simulink library "lib_wheel"  (Simulink 4.1.1)
undefined symbols (not defined in the file or in its folder): veh_mass, wh_axle_loss_mass, wh_axle_loss_trq, wh_front_active_bool, wh_inertia, wh_max_front_brake_force, wh_max_rear_brake_force, wh_radius, wh_rear_active_bool, wh_slip, wh_slip_force_coeff
libraries: lib_wheel x6
(part 1 of 2)
settings Model: LastModifiedBy=tmarkel
settings Model: ModifiedComment=|
  | mokeefe -- Thu Apr 18 08:40:34 2002 -- Version 1.10
  | saving the model:
  | o "without the model browser open"
  | o with only top-level screen visible
  | o with "fit to view" enabled
  | o with "status bar" off and "toolbar" off
  | o with "prompt to update model history with each save" on
settings Model: ModifiedHistory=|
  | mokeefe -- Thu Apr 18 08:40:34 2002 -- Version 1.10
  | saving the model:
  | o "without the model browser open"
  | o with only top-level screen visible
  | o with "fit to view" enabled
  | o with "status bar" off and "toolbar" off
  | o with "prompt to update model history with each save" on
  | 
  | mokeefe -- Thu Apr 18 08:40:34 2002 -- Version 1.10
  | saving the model:
  | o "without the model browser open"
  | o with only top-level screen visible
  | o with "fit to view" enabled
  | o with "status bar" off and "toolbar" off
  | o with "prompt to update model history with each save" on
  | 
  | ssprik -- Fri Feb 01 16:13:25 2002 -- Version 1.9
  | added wheel goto tag wh_trq_a
  | 
  | mokeefe -- Fri Jun 29 14:51:12 2001 -- Version 1.8
  | 
  | added sub-model component to calculate vehicle weight
  | 
  | mokeefe -- Fri Jun 29 14:49:48 2001 -- Version 1.7
  | 
  | 
  | mokeefe -- Thu Jun 28 14:08:49 2001 -- Version 1.6
  | 
  | replaced all 'veh_mass' references with a veh_mass plus a FROM block (originating from drive cycle) that gives variable cargo mass by time

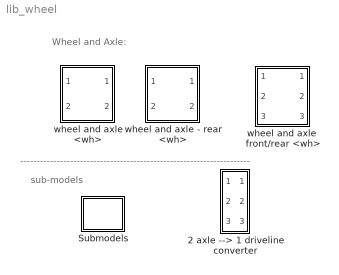
== system lib_wheel ==
  note: Wheel and Axle:
  note: ---------------------------------------------------------------------
  note: sub-models
  2 axle --> 1 driveline converter : Subsystem
      settings: RTWFcnNameOpts=Auto  RTWFileNameOpts=Auto
  Submodels : Subsystem
      settings: RTWFcnNameOpts=Auto  RTWFileNameOpts=Auto
  wheel and axle - rear <wh> : Subsystem
      settings: RTWFcnNameOpts=Auto  RTWFileNameOpts=Auto
      mask Display: image(imread('bdi_wh.jpg'))
  wheel and axle <wh> : Subsystem
      settings: RTWFcnNameOpts=Auto  RTWFileNameOpts=Auto
      mask Display: image(imread('bdi_wh.jpg'))
  wheel and axle  front/rear <wh> : Subsystem
      settings: RTWFcnNameOpts=Auto  RTWFileNameOpts=Auto
      mask Display: image(imread('bdi_wh.jpg'))

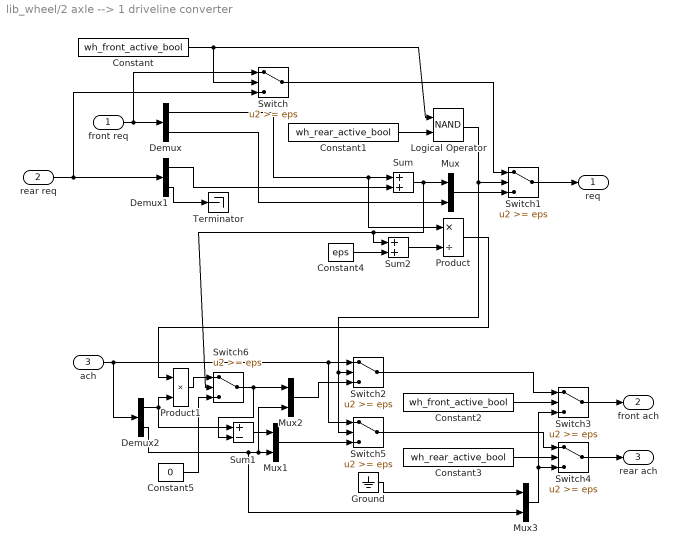
== system lib_wheel/2 axle --> 1 driveline converter ==
  front req : Inport  Port=1  LatchInput=off
  rear req : Inport  Port=2  LatchInput=off
  ach : Inport  Port=3  LatchInput=off
  Constant : Constant  Value=wh_front_active_bool
  Constant1 : Constant  Value=wh_rear_active_bool
  Constant2 : Constant  Value=wh_front_active_bool
  Constant3 : Constant  Value=wh_rear_active_bool
  Constant4 : Constant  Value=eps
  Constant5 : Constant  Value=0
  Demux : Demux  Outputs=2  BusSelectionMode=off
  Demux1 : Demux  Outputs=2  BusSelectionMode=off
  Demux2 : Demux  Outputs=2  BusSelectionMode=off
  Ground : Ground
  Logical Operator : Logic  Operator=NAND  Inputs=2
  Mux{,1..3} (4 alike) : Mux  Inputs=2
  Product : Product  Inputs=*/  Multiplication=Element-wise(.*)  SaturateOnIntegerOverflow=on
  Product1 : Product  Inputs=2  Multiplication=Element-wise(.*)  SaturateOnIntegerOverflow=on
  Sum : Sum  Inputs=++  SaturateOnIntegerOverflow=on
  Sum1 : Sum  Inputs=+-  SaturateOnIntegerOverflow=on
  Sum2 : Sum  Inputs=++  SaturateOnIntegerOverflow=on
  Switch{,1..6} (7 alike) : Switch  Threshold=eps
  Terminator : Terminator
  req : Outport  Port=1
  front ach : Outport  Port=2
  rear ach : Outport  Port=3
  wires:
  rear req/1 -> Demux1/1, Switch/3
  Constant/1 -> Switch/2, Logical Operator/1
  Switch/1 -> Switch1/1
  Logical Operator/1 -> Switch1/2, Switch2/2, Switch5/2
  Switch1/1 -> req/1
  Mux/1 -> Switch1/3
  Demux1/1 -> Sum/2
  Demux/1 -> Sum/1, Product/1
  Sum/1 -> Mux/1, Sum2/1, Switch6/2
  Demux/2 -> Mux/2
  Demux1/2 -> Terminator/1
  front req/1 -> Demux/1, Switch/1
  Constant1/1 -> Logical Operator/2
  ach/1 -> Demux2/1, Switch2/1, Switch5/1
  Switch3/1 -> front ach/1
  Switch4/1 -> rear ach/1
  Demux2/1 -> Product1/2, Sum1/1
  Product/1 -> Product1/1
  Sum1/1 -> Mux1/1
  Constant3/1 -> Switch4/2
  Constant2/1 -> Switch3/2
  Ground/1 -> Mux3/1
  Mux3/1 -> Switch4/3, Switch3/3
  Mux2/1 -> Switch2/3
  Mux1/1 -> Switch5/3
  Switch2/1 -> Switch3/1
  Switch5/1 -> Switch4/1
  Demux2/2 -> Mux1/2, Mux2/2, Mux3/2
  Constant4/1 -> Sum2/2
  Sum2/1 -> Product/2
  Product1/1 -> Switch6/1
  Switch6/1 -> Mux2/1, Sum1/2
  Constant5/1 -> Switch6/3

== system lib_wheel/Submodels ==
  note: vehicle mass calculation (kg)
  veh mass calc : Subsystem
      settings: RTWFcnNameOpts=Auto  RTWFileNameOpts=Auto

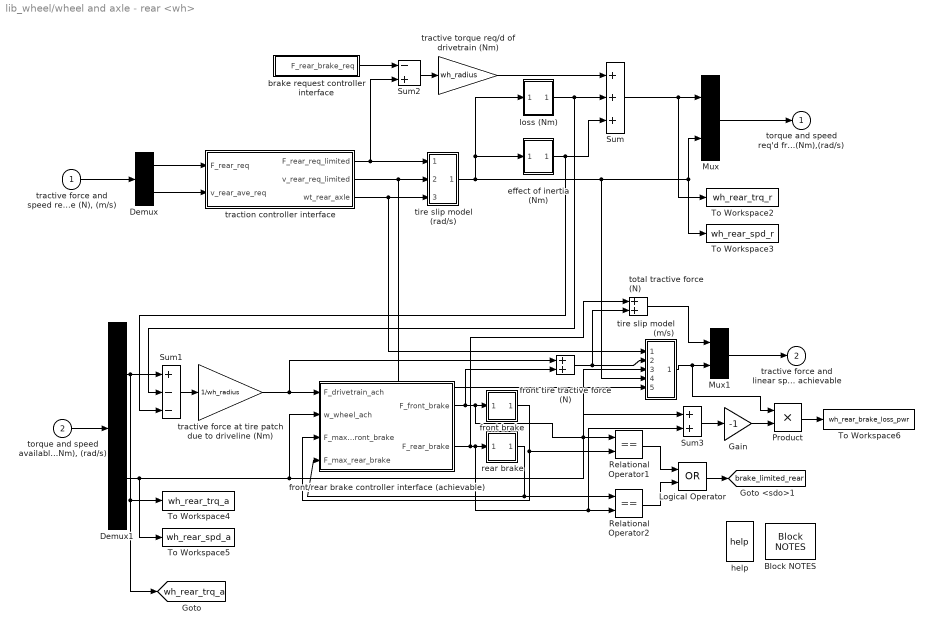
== system lib_wheel/wheel and axle - rear <wh> ==
  "tractive force and speed req'd of tire/road interface (N), (m/s)" : Inport  Port=1  LatchInput=off
  "torque and speed available from drivetrain into axle (Nm), (rad/s)" : Inport  Port=2  LatchInput=off
  Block NOTES : lib_wheel/wheel and axle <wh>/Block NOTES
  Demux : Demux  Outputs=2  BusSelectionMode=off
  Demux1 : Demux  Outputs=2  BusSelectionMode=off
  Gain : Gain  Gain=-1  Multiplication=Element-wise(K.*u)  SaturateOnIntegerOverflow=on
  Logical Operator : Logic  Operator=OR  Inputs=2
  Mux : Mux  Inputs=2
      settings: DisplayOption=none
  Mux1 : Mux  Inputs=2
      settings: DisplayOption=none
  Product : Product  Inputs=2  Multiplication=Element-wise(.*)  SaturateOnIntegerOverflow=on
  Relational Operator1 : RelationalOperator  Operator===
  Relational Operator2 : RelationalOperator  Operator===
  Sum : Sum  Inputs=+++  SaturateOnIntegerOverflow=on
  Sum1 : Sum  Inputs=+--  SaturateOnIntegerOverflow=on
  Sum2 : Sum  Inputs=-+  SaturateOnIntegerOverflow=on
  Sum3 : Sum  Inputs=++  SaturateOnIntegerOverflow=on
  To Workspace2 : ToWorkspace  VariableName=wh_rear_trq_r  SampleTime=-1  SaveFormat=Array
  To Workspace3 : ToWorkspace  VariableName=wh_rear_spd_r  SampleTime=-1  SaveFormat=Array
  To Workspace4 : ToWorkspace  VariableName=wh_rear_trq_a  SampleTime=-1  SaveFormat=Array
  To Workspace5 : ToWorkspace  VariableName=wh_rear_spd_a  SampleTime=-1  SaveFormat=Array
  To Workspace6 : ToWorkspace  VariableName=wh_rear_brake_loss_pwr  SampleTime=-1  SaveFormat=Array
  brake request controller interface : Subsystem
      settings: RTWFcnNameOpts=Auto  RTWFileNameOpts=Auto
  effect of inertia (Nm) : Subsystem
      settings: RTWFcnNameOpts=Auto  RTWFileNameOpts=Auto
  front brake : Subsystem
      settings: RTWFcnNameOpts=Auto  RTWFileNameOpts=Auto
  front tire tractive force (N) : Sum  Inputs=++  SaturateOnIntegerOverflow=on
  front/rear brake controller interface (achievable) : Subsystem
      settings: RTWFcnNameOpts=Auto  RTWFileNameOpts=Auto
  help : lib_wheel/wheel and axle <wh>/help
  loss (Nm) : Subsystem
      settings: RTWFcnNameOpts=Auto  RTWFileNameOpts=Auto
  rear brake : Subsystem
      settings: RTWFcnNameOpts=Auto  RTWFileNameOpts=Auto
  tire slip model (m/s) : Subsystem
      settings: RTWFcnNameOpts=Auto  RTWFileNameOpts=Auto
  tire slip model (rad/s) : Subsystem
      settings: RTWFcnNameOpts=Auto  RTWFileNameOpts=Auto
  total tractive force (N) : Sum  Inputs=++  SaturateOnIntegerOverflow=on
  traction controller interface : Subsystem
      settings: RTWFcnNameOpts=Auto  RTWFileNameOpts=Auto
  tractive force at tire patch due to driveline (Nm) : Gain  Gain=1/wh_radius  Multiplication=Element-wise(K.*u)  SaturateOnIntegerOverflow=on
  tractive torque req/d of drivetrain (Nm) : Gain  Gain=wh_radius  Multiplication=Element-wise(K.*u)  SaturateOnIntegerOverflow=on
  torque and speed req'd from drivetrain into axle (Nm),(rad/s) : Outport  Port=1  InitialOutput=0
  tractive force and linear speed achievable : Outport  Port=2  InitialOutput=0
  tag scope: brake_limited_rear=global, wh_rear_trq_a=global
  wires:
  Demux/1 -> traction controller interface/1(F_rear_req)
  front/rear brake controller interface (achievable)/2(F_rear_brake) -> rear brake/1(F_brake), Relational Operator2/2, Sum3/2, total tractive force (N)/1
  Sum2/1 -> tractive torque req/d of drivetrain (Nm)/1
  traction controller interface/1(F_rear_req_limited) -> Sum2/2, tire slip model (rad/s)/1(tractive force requested of rear axle (N))
  Demux1/2 -> To Workspace5/1, tire slip model (m/s)/3(axle speed available (rad/s)), front/rear brake controller interface (achievable)/2(w_wheel_ach)
  Demux1/1 -> Sum1/1, To Workspace4/1, [wh_rear_trq_a]
  Sum/1 -> To Workspace2/1, Mux/1
  Mux/1 -> torque and speed req'd from drivetrain into axle (Nm),(rad/s)/1
  traction controller interface/3(wt_rear_axle) -> tire slip model (rad/s)/3(weight borne by rear axle (N)), tire slip model (m/s)/1(weight borne by rear axle (N))
  rear brake/1(F_brake_max) -> Relational Operator2/1, front/rear brake controller interface (achievable)/4(F_max_rear_brake)
  front brake/1(F_brake_max) -> Relational Operator1/2, front/rear brake controller interface (achievable)/3(F_max_front_brake)
  front tire tractive force (N)/1 -> total tractive force (N)/2, tire slip model (m/s)/2(tractive force available at rear axle (N))
  front/rear brake controller interface (achievable)/1(F_front_brake) -> front brake/1(F_brake), Relational Operator1/1, Sum3/1, front tire tractive force (N)/2
  brake request controller interface/1(F_rear_brake_req) -> Sum2/1
  "torque and speed available from drivetrain into axle (Nm), (rad/s)"/1 -> Demux1/1
  total tractive force (N)/1 -> Mux1/1
  Mux1/1 -> tractive force and linear speed achievable/1
  tractive torque req/d of drivetrain (Nm)/1 -> Sum/1
  tire slip model (rad/s)/1(slip-augmented rotational speed (rad/s)) -> To Workspace3/1, Mux/2, tire slip model (m/s)/4(axle speed req'd (rad/s)), loss (Nm)/1(axle speed (rad/s)), effect of inertia (Nm)/1(axle input speed (rad/s))
  "tractive force and speed req'd of tire/road interface (N), (m/s)"/1 -> Demux/1
  loss (Nm)/1(drag torque (Nm)) -> Sum1/2, Sum/2
  effect of inertia (Nm)/1(inertia torque (Nm)) -> Sum1/3, Sum/3
  Sum1/1 -> tractive force at tire patch due to driveline (Nm)/1
  tractive force at tire patch due to driveline (Nm)/1 -> front tire tractive force (N)/1, front/rear brake controller interface (achievable)/1(F_drivetrain_ach)
  Relational Operator2/1 -> Logical Operator/2
  Relational Operator1/1 -> Logical Operator/1
  Logical Operator/1 -> [brake_limited_rear]
  Product/1 -> To Workspace6/1
  Sum3/1 -> Gain/1
  Gain/1 -> Product/2
  tire slip model (m/s)/1(possible vehicle speed (m/s)) -> Mux1/2, Product/1
  Demux/2 -> traction controller interface/2(v_rear_ave_req)
  traction controller interface/2(v_rear_req_limited) -> tire slip model (rad/s)/2(requested time-step average vehicle speed (m/s)), tire slip model (m/s)/5(vehicle speed required (m/s))

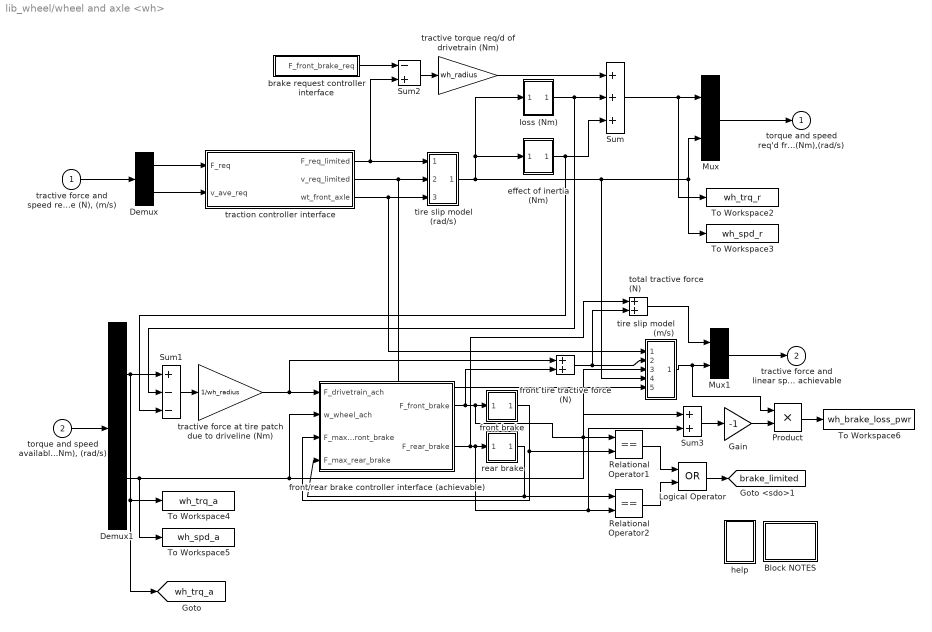
== system lib_wheel/wheel and axle <wh> ==
  "tractive force and speed req'd of tire/road interface (N), (m/s)" : Inport  Port=1  LatchInput=off
  "torque and speed available from drivetrain into axle (Nm), (rad/s)" : Inport  Port=2  LatchInput=off
  Block NOTES : Subsystem
      settings: RTWFcnNameOpts=Auto  RTWFileNameOpts=Auto
      mask Display: disp('Block\nNOTES')
  Demux : Demux  Outputs=2  BusSelectionMode=off
  Demux1 : Demux  Outputs=2  BusSelectionMode=off
  Gain : Gain  Gain=-1  Multiplication=Element-wise(K.*u)  SaturateOnIntegerOverflow=on
  Logical Operator : Logic  Operator=OR  Inputs=2
  Mux : Mux  Inputs=2
      settings: DisplayOption=none
  Mux1 : Mux  Inputs=2
      settings: DisplayOption=none
  Product : Product  Inputs=2  Multiplication=Element-wise(.*)  SaturateOnIntegerOverflow=on
  Relational Operator1 : RelationalOperator  Operator===
  Relational Operator2 : RelationalOperator  Operator===
  Sum : Sum  Inputs=+++  SaturateOnIntegerOverflow=on
  Sum1 : Sum  Inputs=+--  SaturateOnIntegerOverflow=on
  Sum2 : Sum  Inputs=-+  SaturateOnIntegerOverflow=on
  Sum3 : Sum  Inputs=++  SaturateOnIntegerOverflow=on
  To Workspace2 : ToWorkspace  VariableName=wh_trq_r  SampleTime=-1  SaveFormat=Array
  To Workspace3 : ToWorkspace  VariableName=wh_spd_r  SampleTime=-1  SaveFormat=Array
  To Workspace4 : ToWorkspace  VariableName=wh_trq_a  SampleTime=-1  SaveFormat=Array
  To Workspace5 : ToWorkspace  VariableName=wh_spd_a  SampleTime=-1  SaveFormat=Array
  To Workspace6 : ToWorkspace  VariableName=wh_brake_loss_pwr  SampleTime=-1  SaveFormat=Array
  brake request controller interface : Subsystem
      settings: RTWFcnNameOpts=Auto  RTWFileNameOpts=Auto
  effect of inertia (Nm) : Subsystem
      settings: RTWFcnNameOpts=Auto  RTWFileNameOpts=Auto
  front brake : Subsystem
      settings: RTWFcnNameOpts=Auto  RTWFileNameOpts=Auto
  front tire tractive force (N) : Sum  Inputs=++  SaturateOnIntegerOverflow=on
  front/rear brake controller interface (achievable) : Subsystem
      settings: RTWFcnNameOpts=Auto  RTWFileNameOpts=Auto
  help : Subsystem
      settings: OpenFcn=web(['file:\\\' which('advisor_doc.htm')]);  RTWFcnNameOpts=Auto  RTWFileNameOpts=Auto
      mask Display: image(imread('doc_man.jpg'))
  loss (Nm) : Subsystem
      settings: RTWFcnNameOpts=Auto  RTWFileNameOpts=Auto
  rear brake : Subsystem
      settings: RTWFcnNameOpts=Auto  RTWFileNameOpts=Auto
  tire slip model (m/s) : Subsystem
      settings: RTWFcnNameOpts=Auto  RTWFileNameOpts=Auto
  tire slip model (rad/s) : Subsystem
      settings: RTWFcnNameOpts=Auto  RTWFileNameOpts=Auto
  total tractive force (N) : Sum  Inputs=++  SaturateOnIntegerOverflow=on
  traction controller interface : Subsystem
      settings: RTWFcnNameOpts=Auto  RTWFileNameOpts=Auto
  tractive force at tire patch due to driveline (Nm) : Gain  Gain=1/wh_radius  Multiplication=Element-wise(K.*u)  SaturateOnIntegerOverflow=on
  tractive torque req/d of drivetrain (Nm) : Gain  Gain=wh_radius  Multiplication=Element-wise(K.*u)  SaturateOnIntegerOverflow=on
  torque and speed req'd from drivetrain into axle (Nm),(rad/s) : Outport  Port=1  InitialOutput=0
  tractive force and linear speed achievable : Outport  Port=2  InitialOutput=0
  tag scope: brake_limited=global, wh_trq_a=global
  wires:
  Demux/1 -> traction controller interface/1(F_req)
  front/rear brake controller interface (achievable)/2(F_rear_brake) -> rear brake/1(F_brake), Relational Operator2/2, Sum3/2, total tractive force (N)/1
  Sum2/1 -> tractive torque req/d of drivetrain (Nm)/1
  traction controller interface/1(F_req_limited) -> tire slip model (rad/s)/1(tractive force requested of front axle (N)), Sum2/2
  Demux1/2 -> To Workspace5/1, tire slip model (m/s)/3(axle speed available (rad/s)), front/rear brake controller interface (achievable)/2(w_wheel_ach)
  Demux1/1 -> Sum1/1, To Workspace4/1, [wh_trq_a]
  Sum/1 -> To Workspace2/1, Mux/1
  Mux/1 -> torque and speed req'd from drivetrain into axle (Nm),(rad/s)/1
  traction controller interface/3(wt_front_axle) -> tire slip model (m/s)/1(weight borne by front axle (N)), tire slip model (rad/s)/3(weight borne by front axle (N))
  rear brake/1(F_brake_max) -> Relational Operator2/1, front/rear brake controller interface (achievable)/4(F_max_rear_brake)
  front brake/1(F_brake_max) -> Relational Operator1/2, front/rear brake controller interface (achievable)/3(F_max_front_brake)
  front tire tractive force (N)/1 -> tire slip model (m/s)/2(tractive force available at front axle (N)), total tractive force (N)/2
  front/rear brake controller interface (achievable)/1(F_front_brake) -> front brake/1(F_brake), Relational Operator1/1, Sum3/1, front tire tractive force (N)/2
  brake request controller interface/1(F_front_brake_req) -> Sum2/1
  "torque and speed available from drivetrain into axle (Nm), (rad/s)"/1 -> Demux1/1
  total tractive force (N)/1 -> Mux1/1
  Mux1/1 -> tractive force and linear speed achievable/1
  tractive torque req/d of drivetrain (Nm)/1 -> Sum/1
  tire slip model (rad/s)/1(slip-augmented rotational speed (rad/s)) -> tire slip model (m/s)/4(axle speed req'd (rad/s)), To Workspace3/1, Mux/2, loss (Nm)/1(axle speed (rad/s)), effect of inertia (Nm)/1(axle input speed (rad/s))
  "tractive force and speed req'd of tire/road interface (N), (m/s)"/1 -> Demux/1
  loss (Nm)/1(drag torque (Nm)) -> Sum1/2, Sum/2
  effect of inertia (Nm)/1(inertia torque (Nm)) -> Sum1/3, Sum/3
  Sum1/1 -> tractive force at tire patch due to driveline (Nm)/1
  tractive force at tire patch due to driveline (Nm)/1 -> front tire tractive force (N)/1, front/rear brake controller interface (achievable)/1(F_drivetrain_ach)
  Relational Operator2/1 -> Logical Operator/2
  Relational Operator1/1 -> Logical Operator/1
  Logical Operator/1 -> [brake_limited]
  Product/1 -> To Workspace6/1
  Sum3/1 -> Gain/1
  Gain/1 -> Product/2
  tire slip model (m/s)/1(possible vehicle speed (m/s)) -> Mux1/2, Product/1
  Demux/2 -> traction controller interface/2(v_ave_req)
  traction controller interface/2(v_req_limited) -> tire slip model (m/s)/5(vehicle speed required (m/s)), tire slip model (rad/s)/2(requested time-step average vehicle speed (m/s))

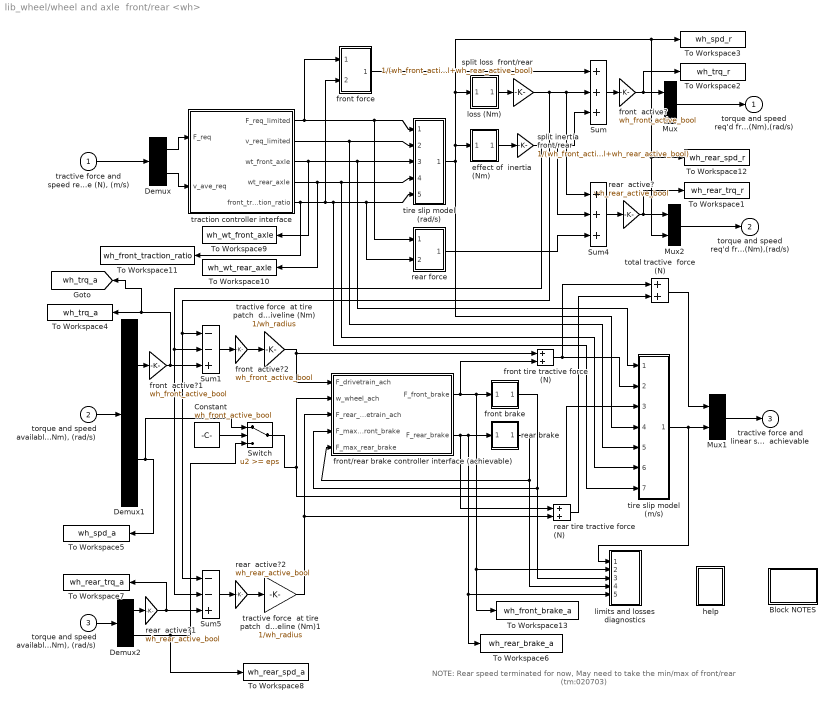
== system lib_wheel/wheel and axle  front/rear <wh> ==
  note: NOTE: Rear speed terminated for now, May need to take the min/max of front/rear (tm:020703)
  "tractive force and speed req'd of tire/road interface (N), (m/s)" : Inport  Port=1  LatchInput=off
  "torque and speed available from drivetrain into front axle (Nm), (rad/s)" : Inport  Port=2  LatchInput=off
  "torque and speed available from drivetrain into rear axle (Nm), (rad/s)" : Inport  Port=3  LatchInput=off
  Block NOTES : Subsystem
      settings: RTWFcnNameOpts=Auto  RTWFileNameOpts=Auto
      mask Display: disp('Block\nNOTES')
  Constant : Constant  Value=wh_front_active_bool
  Demux : Demux  Outputs=2  BusSelectionMode=off
  Demux1 : Demux  Outputs=2  BusSelectionMode=off
  Demux2 : Demux  Outputs=2  BusSelectionMode=off
  Mux : Mux  Inputs=2
      settings: DisplayOption=none
  Mux1 : Mux  Inputs=2
      settings: DisplayOption=none
  Mux2 : Mux  Inputs=2
      settings: DisplayOption=none
  Sum : Sum  Inputs=+++  SaturateOnIntegerOverflow=on
  Sum1 : Sum  Inputs=--+  SaturateOnIntegerOverflow=on
  Sum4 : Sum  Inputs=+++  SaturateOnIntegerOverflow=on
  Sum5 : Sum  Inputs=--+  SaturateOnIntegerOverflow=on
  Switch : Switch  Threshold=eps
  To Workspace1 : ToWorkspace  VariableName=wh_rear_trq_r  SampleTime=-1  SaveFormat=Array
  To Workspace10 : ToWorkspace  VariableName=wh_wt_rear_axle  SampleTime=-1  SaveFormat=Array
  To Workspace11 : ToWorkspace  VariableName=wh_front_traction_ratio  SampleTime=-1  SaveFormat=Array
  To Workspace12 : ToWorkspace  VariableName=wh_rear_spd_r  SampleTime=-1  SaveFormat=Array
  To Workspace13 : ToWorkspace  VariableName=wh_front_brake_a  SampleTime=-1  SaveFormat=Array
  To Workspace2 : ToWorkspace  VariableName=wh_trq_r  SampleTime=-1  SaveFormat=Array
  To Workspace3 : ToWorkspace  VariableName=wh_spd_r  SampleTime=-1  SaveFormat=Array
  To Workspace4 : ToWorkspace  VariableName=wh_trq_a  SampleTime=-1  SaveFormat=Array
  To Workspace5 : ToWorkspace  VariableName=wh_spd_a  SampleTime=-1  SaveFormat=Array
  To Workspace6 : ToWorkspace  VariableName=wh_rear_brake_a  SampleTime=-1  SaveFormat=Array
  To Workspace7 : ToWorkspace  VariableName=wh_rear_trq_a  SampleTime=-1  SaveFormat=Array
  To Workspace8 : ToWorkspace  VariableName=wh_rear_spd_a  SampleTime=-1  SaveFormat=Array
  To Workspace9 : ToWorkspace  VariableName=wh_wt_front_axle  SampleTime=-1  SaveFormat=Array
  effect of  inertia (Nm) : Subsystem
      settings: RTWFcnNameOpts=Auto  RTWFileNameOpts=Auto
  front  active? : Gain  Gain=wh_front_active_bool  Multiplication=Element-wise(K.*u)  SaturateOnIntegerOverflow=on
  front  active?1 : Gain  Gain=wh_front_active_bool  Multiplication=Element-wise(K.*u)  SaturateOnIntegerOverflow=on
  front  active?2 : Gain  Gain=wh_front_active_bool  Multiplication=Element-wise(K.*u)  SaturateOnIntegerOverflow=on
  front brake : Subsystem
      settings: RTWFcnNameOpts=Auto  RTWFileNameOpts=Auto
  front force : Subsystem
      settings: RTWFcnNameOpts=Auto  RTWFileNameOpts=Auto
  front tire tractive force (N) : Sum  Inputs=++  SaturateOnIntegerOverflow=on
  front/rear brake controller interface (achievable) : Subsystem
      settings: RTWFcnNameOpts=Auto  RTWFileNameOpts=Auto
  help : Subsystem
      settings: OpenFcn=web(['file:\\\' which('advisor_doc.htm')]);  RTWFcnNameOpts=Auto  RTWFileNameOpts=Auto
      mask Display: image(imread('doc_man.jpg'))
  limits and losses diagnostics : Subsystem
      settings: RTWFcnNameOpts=Auto  RTWFileNameOpts=Auto
  loss (Nm) : Subsystem
      settings: RTWFcnNameOpts=Auto  RTWFileNameOpts=Auto
  rear  active? : Gain  Gain=wh_rear_active_bool  Multiplication=Element-wise(K.*u)  SaturateOnIntegerOverflow=on
  rear  active?1 : Gain  Gain=wh_rear_active_bool  Multiplication=Element-wise(K.*u)  SaturateOnIntegerOverflow=on
  rear  active?2 : Gain  Gain=wh_rear_active_bool  Multiplication=Element-wise(K.*u)  SaturateOnIntegerOverflow=on
  rear brake : Subsystem
      settings: RTWFcnNameOpts=Auto  RTWFileNameOpts=Auto
  rear force : Subsystem
      settings: RTWFcnNameOpts=Auto  RTWFileNameOpts=Auto
  rear tire tractive force (N) : Sum  Inputs=++  SaturateOnIntegerOverflow=on
  split inertia front/rear : Gain  Gain=1/(wh_front_active_bool+wh_rear_active_bool)  Multiplication=Element-wise(K.*u)  SaturateOnIntegerOverflow=on
  split loss  front/rear : Gain  Gain=1/(wh_front_active_bool+wh_rear_active_bool)  Multiplication=Element-wise(K.*u)  SaturateOnIntegerOverflow=on
  tire slip model (m/s) : Subsystem
      settings: RTWFcnNameOpts=Auto  RTWFileNameOpts=Auto
  tire slip model (rad/s) : Subsystem
      settings: RTWFcnNameOpts=Auto  RTWFileNameOpts=Auto
  total tractive  force (N) : Sum  Inputs=++  SaturateOnIntegerOverflow=on
  traction controller interface : Subsystem
      settings: RTWFcnNameOpts=Auto  RTWFileNameOpts=Auto
  tractive force  at tire patch  due to driveline (Nm) : Gain  Gain=1/wh_radius  Multiplication=Element-wise(K.*u)  SaturateOnIntegerOverflow=on
  tractive force  at tire patch  due to driveline (Nm)1 : Gain  Gain=1/wh_radius  Multiplication=Element-wise(K.*u)  SaturateOnIntegerOverflow=on
  torque and speed req'd from drivetrain into front axle (Nm),(rad/s) : Outport  Port=1  InitialOutput=0
  torque and speed req'd from drivetrain into rear axle (Nm),(rad/s) : Outport  Port=2  InitialOutput=0
  tractive force and linear speed  achievable : Outport  Port=3  InitialOutput=0
  tag scope: wh_trq_a=global
  wires:
  traction controller interface/2(v_req_limited) -> tire slip model (rad/s)/2(requested time-step average vehicle speed (m/s)), tire slip model (m/s)/5(vehicle speed required (m/s))
  Demux/2 -> traction controller interface/2(v_ave_req)
  tire slip model (m/s)/1(possible vehicle speed (m/s)) -> Mux1/2, limits and losses diagnostics/1(speed)
  tractive force  at tire patch  due to driveline (Nm)/1 -> front/rear brake controller interface (achievable)/1(F_drivetrain_ach), front tire tractive force (N)/1
  Sum1/1 -> front  active?2/1
  effect of  inertia (Nm)/1(inertia torque (Nm)) -> split inertia front/rear/1
  loss (Nm)/1(drag torque (Nm)) -> split loss  front/rear/1
  "tractive force and speed req'd of tire/road interface (N), (m/s)"/1 -> Demux/1
  tire slip model (rad/s)/1(slip-augmented rotational speed (rad/s)) -> effect of  inertia (Nm)/1(axle input speed (rad/s)), loss (Nm)/1(axle speed (rad/s)), To Workspace3/1, Mux/2, Mux2/2, To Workspace12/1, tire slip model (m/s)/4(axle speed req'd (rad/s))
  front force/1(Out1) -> Sum/1
  Mux1/1 -> tractive force and linear speed  achievable/1
  total tractive  force (N)/1 -> Mux1/1
  "torque and speed available from drivetrain into front axle (Nm), (rad/s)"/1 -> Demux1/1
  front/rear brake controller interface (achievable)/1(F_front_brake) -> front tire tractive force (N)/2, front brake/1(F_brake), limits and losses diagnostics/2(front brake), To Workspace13/1
  front tire tractive force (N)/1 -> tire slip model (m/s)/2(total tractive  force available (N)), total tractive  force (N)/1
  front brake/1(F_brake_max) -> front/rear brake controller interface (achievable)/4(F_max_front_brake), limits and losses diagnostics/3(front brake max)
  rear brake/1(F_brake_max) -> front/rear brake controller interface (achievable)/5(F_max_rear_brake), limits and losses diagnostics/4(rear brake max)
  traction controller interface/3(wt_front_axle) -> tire slip model (rad/s)/3(weight borne by front axle (N)), tire slip model (m/s)/1(weight borne  by front axle (N)), To Workspace9/1
  Mux/1 -> torque and speed req'd from drivetrain into front axle (Nm),(rad/s)/1
  Sum/1 -> front  active?/1
  Demux1/1 -> front  active?1/1
  Switch/1 -> front/rear brake controller interface (achievable)/2(w_wheel_ach), tire slip model (m/s)/3(axle speed available (rad/s))
  traction controller interface/1(F_req_limited) -> rear force/1(In1), tire slip model (rad/s)/1(total tractive  force requested (N)), front force/1(In1)
  front/rear brake controller interface (achievable)/2(F_rear_brake) -> rear tire tractive force (N)/1, rear brake/1(F_brake), limits and losses diagnostics/5(rear brake), To Workspace6/1
  Demux/1 -> traction controller interface/1(F_req)
  traction controller interface/5(front_traction_ratio) -> tire slip model (m/s)/7(front fraction), tire slip model (rad/s)/5(front traction ratio), rear force/2(In2), front force/2(In2), To Workspace11/1
  rear force/1(Out1) -> Sum4/3
  Sum4/1 -> rear  active?/1
  Mux2/1 -> torque and speed req'd from drivetrain into rear axle (Nm),(rad/s)/1
  split loss  front/rear/1 -> Sum/2, Sum4/1, Sum1/1, Sum5/1
  split inertia front/rear/1 -> Sum/3, Sum4/2, Sum1/2, Sum5/2
  traction controller interface/4(wt_rear_axle) -> tire slip model (rad/s)/4(weight borne by  rear axle (N)1), tire slip model (m/s)/6(weight borne by  rear axle (N)), To Workspace10/1
  Sum5/1 -> rear  active?2/1
  "torque and speed available from drivetrain into rear axle (Nm), (rad/s)"/1 -> Demux2/1
  tractive force  at tire patch  due to driveline (Nm)1/1 -> front/rear brake controller interface (achievable)/3(F_rear_drivetrain_ach), rear tire tractive force (N)/2
  rear tire tractive force (N)/1 -> total tractive  force (N)/2
  Demux2/1 -> rear  active?1/1
  Demux2/2 -> To Workspace8/1, Switch/3
  front  active?/1 -> Mux/1, To Workspace2/1
  rear  active?/1 -> To Workspace1/1, Mux2/1
  front  active?1/1 -> To Workspace4/1, [wh_trq_a], Sum1/3
  rear  active?1/1 -> To Workspace7/1, Sum5/3
  rear  active?2/1 -> tractive force  at tire patch  due to driveline (Nm)1/1
  front  active?2/1 -> tractive force  at tire patch  due to driveline (Nm)/1
  Constant/1 -> Switch/2
  Demux1/2 -> Switch/1, To Workspace5/1

== system lib_wheel/Submodels/veh mass calc ==
  Constant : Constant  Value=veh_mass
  Sum : Sum  Inputs=|++  SaturateOnIntegerOverflow=on
  Out1 : Outport  Port=1
  wires:
  [veh_cargo_mass] -> Sum/1
  Constant/1 -> Sum/2
  Sum/1 -> Out1/1

== system lib_wheel/wheel and axle - rear <wh>/brake request controller interface ==
  F_rear_brake_req : Outport  Port=1  InitialOutput=0
  wires:
  [F_rear_brake_req] -> F_rear_brake_req/1

== system lib_wheel/wheel and axle - rear <wh>/effect of inertia (Nm) ==
  note: This block computes the torque required to overcome the inertia of the
      | wheels and axle.
  axle input speed (rad/s) : Inport  Port=1  LatchInput=off
  Constant : Constant  Value=wh_inertia
  Product : Product  Inputs=2  Multiplication=Element-wise(.*)  SaturateOnIntegerOverflow=on
  d/dt : Derivative
  inertia torque (Nm) : Outport  Port=1  InitialOutput=0
  wires:
  d/dt/1 -> Product/1
  axle input speed (rad/s)/1 -> d/dt/1
  Constant/1 -> Product/2
  Product/1 -> inertia torque (Nm)/1

== system lib_wheel/wheel and axle - rear <wh>/front brake ==
  F_brake : Inport  Port=1  LatchInput=off
  Constant : Constant  Value=-inf
  Terminator : Terminator
  F_brake_max : Outport  Port=1  InitialOutput=0
  wires:
  F_brake/1 -> Terminator/1
  Constant/1 -> F_brake_max/1

== system lib_wheel/wheel and axle - rear <wh>/front/rear brake controller interface (achievable) ==
  F_drivetrain_ach : Inport  Port=1  LatchInput=off
  w_wheel_ach : Inport  Port=2  LatchInput=off
  F_max_front_brake : Inport  Port=3  LatchInput=off
  F_max_rear_brake : Inport  Port=4  LatchInput=off
  F_front_brake : Outport  Port=1  InitialOutput=0
  F_rear_brake : Outport  Port=2  InitialOutput=0
  tag scope: F_drivetrain_ach=global, F_max_front_brake=global, F_max_rear_brake=global, w_wheel_ach=global
  wires:
  F_max_rear_brake/1 -> [F_max_rear_brake]
  F_max_front_brake/1 -> [F_max_front_brake]
  F_drivetrain_ach/1 -> [F_drivetrain_ach]
  w_wheel_ach/1 -> [w_wheel_ach]
  [F_front_brake] -> F_front_brake/1
  [F_rear_brake] -> F_rear_brake/1

== system lib_wheel/wheel and axle - rear <wh>/loss (Nm) ==
  note: The loss torque is zero when the axle is not turning.
  axle speed (rad/s) : Inport  Port=1  LatchInput=off
  Constant : Constant  Orientation=up  Value=0
  Switch : Switch  Threshold=eps
  veh mass calc : lib_wheel/Submodels/veh mass calc
      settings: RTWFcnNameOpts=Auto  RTWFileNameOpts=Auto
  wheel & axle bearing drag (Nm) : Lookup  InputValues=wh_axle_loss_mass  OutputValues=wh_axle_loss_trq
  drag torque (Nm) : Outport  Port=1  InitialOutput=0
  wires:
  veh mass calc/1 -> wheel & axle bearing drag (Nm)/1
  Switch/1 -> drag torque (Nm)/1
  axle speed (rad/s)/1 -> Switch/2
  Constant/1 -> Switch/3
  wheel & axle bearing drag (Nm)/1 -> Switch/1

== system lib_wheel/wheel and axle - rear <wh>/rear brake ==
  F_brake : Inport  Port=1  LatchInput=off
  Constant : Constant  Value=-inf
  Terminator : Terminator
  F_brake_max : Outport  Port=1  InitialOutput=0
  wires:
  Constant/1 -> F_brake_max/1
  F_brake/1 -> Terminator/1

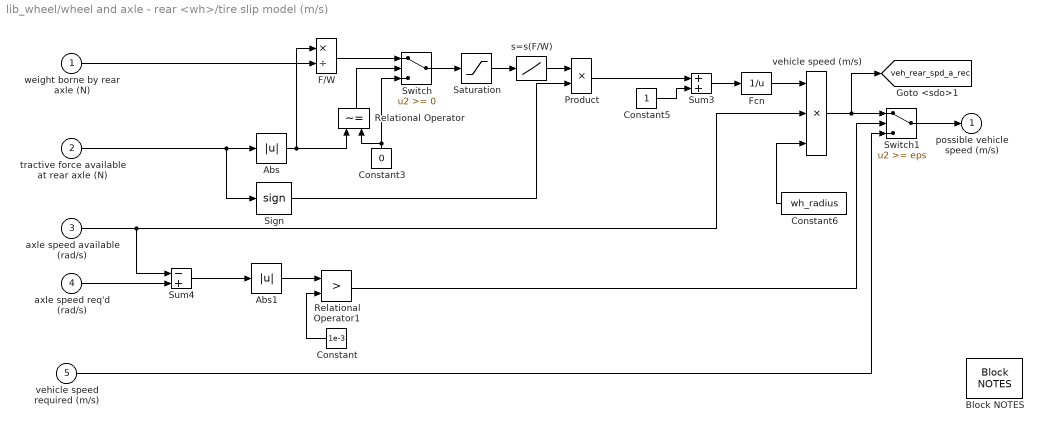
== system lib_wheel/wheel and axle - rear <wh>/tire slip model (m/s) ==
  weight borne by rear axle (N) : Inport  Port=1  LatchInput=off
  tractive force available at rear axle (N) : Inport  Port=2  LatchInput=off
  axle speed available (rad/s) : Inport  Port=3  LatchInput=off
  axle speed req'd (rad/s) : Inport  Port=4  LatchInput=off
  vehicle speed required (m/s) : Inport  Port=5  LatchInput=off
  Abs : Abs  SaturateOnIntegerOverflow=on
  Abs1 : Abs  SaturateOnIntegerOverflow=on
  Block NOTES : lib_wheel/wheel and axle <wh>/tire slip model (m//s)/Block NOTES
  Constant : Constant  Orientation=left  Value=1e-3
  Constant3 : Constant  Orientation=up  Value=0
  Constant5 : Constant  Value=1
  Constant6 : Constant  Orientation=left  Value=wh_radius
  F/W : Product  Inputs=*/  Multiplication=Element-wise(.*)  SaturateOnIntegerOverflow=on
  Fcn : Fcn  Expr=1/u
  Product : Product  Inputs=2  Multiplication=Element-wise(.*)  SaturateOnIntegerOverflow=on
  Relational Operator : RelationalOperator  Orientation=up  Operator=~=
  Relational Operator1 : RelationalOperator  Operator=>
  Saturation : Saturate  UpperLimit=max(wh_slip_force_coeff)  LowerLimit=min(wh_slip_force_coeff)  LinearizeAsGain=on
  Sign : Signum
  Sum3 : Sum  Inputs=++  SaturateOnIntegerOverflow=on
  Sum4 : Sum  Inputs=-+  SaturateOnIntegerOverflow=on
  Switch : Switch  Threshold=0
  Switch1 : Switch  Threshold=eps
  s=s(F/W) : Lookup  InputValues=wh_slip_force_coeff  OutputValues=wh_slip
  vehicle speed (m/s) : Product  Inputs=3  Multiplication=Element-wise(.*)  SaturateOnIntegerOverflow=on
  possible vehicle speed (m/s) : Outport  Port=1  InitialOutput=0
  tag scope: veh_rear_spd_a_rec=global
  wires:
  Product/1 -> Sum3/1
  vehicle speed (m/s)/1 -> [veh_rear_spd_a_rec], Switch1/1
  Switch1/1 -> possible vehicle speed (m/s)/1
  tractive force available at rear axle (N)/1 -> Abs/1, Sign/1
  weight borne by rear axle (N)/1 -> F/W/2
  Abs1/1 -> Relational Operator1/1
  Constant/1 -> Relational Operator1/2
  axle speed req'd (rad/s)/1 -> Sum4/2
  Sum4/1 -> Abs1/1
  vehicle speed required (m/s)/1 -> Switch1/3
  Relational Operator1/1 -> Switch1/2
  Constant6/1 -> vehicle speed (m/s)/3
  axle speed available (rad/s)/1 -> vehicle speed (m/s)/2, Sum4/1
  s=s(F/W)/1 -> Product/1
  Sign/1 -> Product/2
  F/W/1 -> Switch/1
  Constant5/1 -> Sum3/2
  Fcn/1 -> vehicle speed (m/s)/1
  Sum3/1 -> Fcn/1
  Switch/1 -> Saturation/1
  Saturation/1 -> s=s(F/W)/1
  Abs/1 -> Relational Operator/1, F/W/1
  Relational Operator/1 -> Switch/2
  Constant3/1 -> Relational Operator/2, Switch/3

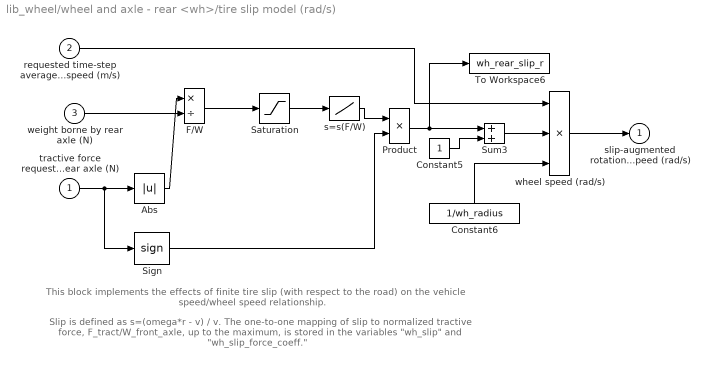
== system lib_wheel/wheel and axle - rear <wh>/tire slip model (rad/s) ==
  note: This block implements the effects of finite tire slip
      | (with respect to the road) on the vehicle speed/wheel speed relationship.
  note: Slip is defined as s=(omega*r - v) / v.  The one-to-one mapping of slip to normalized
      | tractive force, F_tract/W_front_axle, up to the maximum, is stored in the variables
      | "wh_slip" and "wh_slip_force_coeff."
  tractive force requested of rear axle (N) : Inport  Port=1  LatchInput=off
  requested time-step average vehicle speed (m/s) : Inport  Port=2  LatchInput=off
  weight borne by rear axle (N) : Inport  Port=3  LatchInput=off
  Abs : Abs  SaturateOnIntegerOverflow=on
  Constant5 : Constant  Value=1
  Constant6 : Constant  Orientation=up  Value=1/wh_radius
  F/W : Product  Inputs=*/  Multiplication=Element-wise(.*)  SaturateOnIntegerOverflow=on
  Product : Product  Inputs=2  Multiplication=Element-wise(.*)  SaturateOnIntegerOverflow=on
  Saturation : Saturate  UpperLimit=max(wh_slip_force_coeff)  LowerLimit=min(wh_slip_force_coeff)  LinearizeAsGain=on
  Sign : Signum
  Sum3 : Sum  Inputs=++  SaturateOnIntegerOverflow=on
  To Workspace6 : ToWorkspace  VariableName=wh_rear_slip_r  SampleTime=-1  SaveFormat=Array
  s=s(F/W) : Lookup  InputValues=wh_slip_force_coeff  OutputValues=wh_slip
  wheel speed (rad/s) : Product  Inputs=3  Multiplication=Element-wise(.*)  SaturateOnIntegerOverflow=on
  slip-augmented rotational speed (rad/s) : Outport  Port=1  InitialOutput=0
  wires:
  Product/1 -> To Workspace6/1, Sum3/1
  s=s(F/W)/1 -> Product/1
  wheel speed (rad/s)/1 -> slip-augmented rotational speed (rad/s)/1
  tractive force requested of rear axle (N)/1 -> Abs/1, Sign/1
  Constant5/1 -> Sum3/2
  Sum3/1 -> wheel speed (rad/s)/2
  Constant6/1 -> wheel speed (rad/s)/3
  requested time-step average vehicle speed (m/s)/1 -> wheel speed (rad/s)/1
  Sign/1 -> Product/2
  Abs/1 -> F/W/1
  F/W/1 -> Saturation/1
  Saturation/1 -> s=s(F/W)/1
  weight borne by rear axle (N)/1 -> F/W/2

== system lib_wheel/wheel and axle - rear <wh>/traction controller interface ==
  F_rear_req : Inport  Port=1  LatchInput=off
  v_rear_ave_req : Inport  Port=2  LatchInput=off
  F_rear_req_limited : Outport  Port=1  InitialOutput=0
  v_rear_req_limited : Outport  Port=2  InitialOutput=0
  wt_rear_axle : Outport  Port=3  InitialOutput=0
  tag scope: F_rear_req=global, v_rear_ave_req=global
  wires:
  [F_rear_req_limited] -> F_rear_req_limited/1
  [v_rear_req_limited] -> v_rear_req_limited/1
  [wt_rear_axle] -> wt_rear_axle/1
  F_rear_req/1 -> [F_rear_req]
  v_rear_ave_req/1 -> [v_rear_ave_req]

== system lib_wheel/wheel and axle <wh>/Block NOTES ==
  note: This block determines the required axle torque and speed given the tractive force and
      | speed required to meet the trace in the top blocks, and determines the available tractive
      | force and possible vehicle speed given the drivetrain-input torque and rotational speed
      | in the bottom blocks.  The "wheel control" blocks apply the braking strategy and ensure
      | that accelerations beyond the capability of the tires are not requested.

== system lib_wheel/wheel and axle <wh>/brake request controller interface ==
  F_front_brake_req : Outport  Port=1  InitialOutput=0
  wires:
  [F_front_brake_req] -> F_front_brake_req/1

== system lib_wheel/wheel and axle <wh>/effect of inertia (Nm) ==
  note: This block computes the torque required to overcome the inertia of the
      | wheels and axle.
  axle input speed (rad/s) : Inport  Port=1  LatchInput=off
  Constant : Constant  Value=wh_inertia
  Product : Product  Inputs=2  Multiplication=Element-wise(.*)  SaturateOnIntegerOverflow=on
  d/dt : Derivative
  inertia torque (Nm) : Outport  Port=1  InitialOutput=0
  wires:
  Product/1 -> inertia torque (Nm)/1
  Constant/1 -> Product/2
  axle input speed (rad/s)/1 -> d/dt/1
  d/dt/1 -> Product/1

== system lib_wheel/wheel and axle <wh>/front brake ==
  F_brake : Inport  Port=1  LatchInput=off
  Constant : Constant  Value=-inf
  Terminator : Terminator
  F_brake_max : Outport  Port=1  InitialOutput=0
  wires:
  Constant/1 -> F_brake_max/1
  F_brake/1 -> Terminator/1

== system lib_wheel/wheel and axle <wh>/front/rear brake controller interface (achievable) ==
  F_drivetrain_ach : Inport  Port=1  LatchInput=off
  w_wheel_ach : Inport  Port=2  LatchInput=off
  F_max_front_brake : Inport  Port=3  LatchInput=off
  F_max_rear_brake : Inport  Port=4  LatchInput=off
  F_front_brake : Outport  Port=1  InitialOutput=0
  F_rear_brake : Outport  Port=2  InitialOutput=0
  tag scope: F_drivetrain_ach=global, F_max_front_brake=global, F_max_rear_brake=global, w_wheel_ach=global
  wires:
  F_max_rear_brake/1 -> [F_max_rear_brake]
  F_max_front_brake/1 -> [F_max_front_brake]
  F_drivetrain_ach/1 -> [F_drivetrain_ach]
  w_wheel_ach/1 -> [w_wheel_ach]
  [F_front_brake] -> F_front_brake/1
  [F_rear_brake] -> F_rear_brake/1

== system lib_wheel/wheel and axle <wh>/help ==

== system lib_wheel/wheel and axle <wh>/loss (Nm) ==
  note: The loss torque is zero when the axle is not turning.
  axle speed (rad/s) : Inport  Port=1  LatchInput=off
  Constant : Constant  Orientation=up  Value=0
  Switch : Switch  Threshold=eps
  veh mass calc : lib_wheel/Submodels/veh mass calc
      settings: RTWFcnNameOpts=Auto  RTWFileNameOpts=Auto
  wheel & axle bearing drag (Nm) : Lookup  InputValues=wh_axle_loss_mass  OutputValues=wh_axle_loss_trq
  drag torque (Nm) : Outport  Port=1  InitialOutput=0
  wires:
  wheel & axle bearing drag (Nm)/1 -> Switch/1
  Constant/1 -> Switch/3
  axle speed (rad/s)/1 -> Switch/2
  Switch/1 -> drag torque (Nm)/1
  veh mass calc/1 -> wheel & axle bearing drag (Nm)/1

== system lib_wheel/wheel and axle <wh>/rear brake ==
  F_brake : Inport  Port=1  LatchInput=off
  Constant : Constant  Value=-inf
  Terminator : Terminator
  F_brake_max : Outport  Port=1  InitialOutput=0
  wires:
  F_brake/1 -> Terminator/1
  Constant/1 -> F_brake_max/1

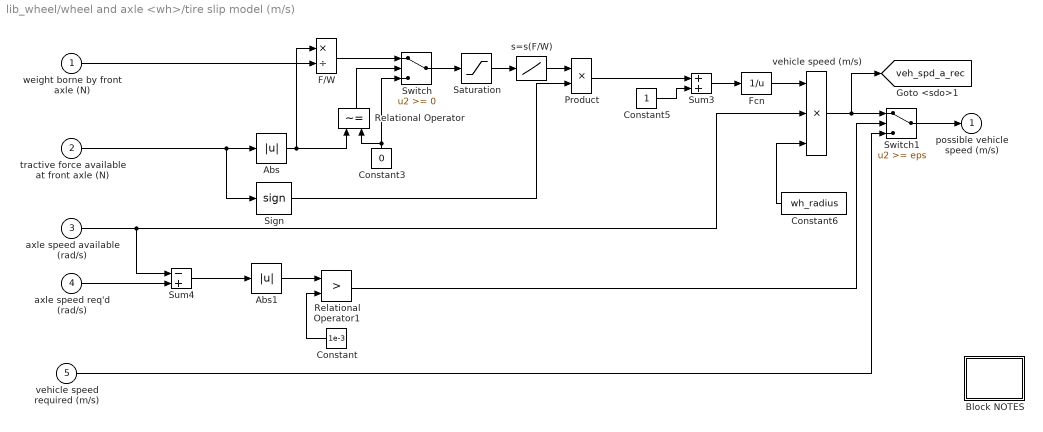
== system lib_wheel/wheel and axle <wh>/tire slip model (m/s) ==
  weight borne by front axle (N) : Inport  Port=1  LatchInput=off
  tractive force available at front axle (N) : Inport  Port=2  LatchInput=off
  axle speed available (rad/s) : Inport  Port=3  LatchInput=off
  axle speed req'd (rad/s) : Inport  Port=4  LatchInput=off
  vehicle speed required (m/s) : Inport  Port=5  LatchInput=off
  Abs : Abs  SaturateOnIntegerOverflow=on
  Abs1 : Abs  SaturateOnIntegerOverflow=on
  Block NOTES : Subsystem
      settings: RTWFcnNameOpts=Auto  RTWFileNameOpts=Auto
      mask Display: disp('Block\nNOTES')
  Constant : Constant  Orientation=left  Value=1e-3
  Constant3 : Constant  Orientation=up  Value=0
  Constant5 : Constant  Value=1
  Constant6 : Constant  Orientation=left  Value=wh_radius
  F/W : Product  Inputs=*/  Multiplication=Element-wise(.*)  SaturateOnIntegerOverflow=on
  Fcn : Fcn  Expr=1/u
  Product : Product  Inputs=2  Multiplication=Element-wise(.*)  SaturateOnIntegerOverflow=on
  Relational Operator : RelationalOperator  Orientation=up  Operator=~=
  Relational Operator1 : RelationalOperator  Operator=>
  Saturation : Saturate  UpperLimit=max(wh_slip_force_coeff)  LowerLimit=min(wh_slip_force_coeff)  LinearizeAsGain=on
  Sign : Signum
  Sum3 : Sum  Inputs=++  SaturateOnIntegerOverflow=on
  Sum4 : Sum  Inputs=-+  SaturateOnIntegerOverflow=on
  Switch : Switch  Threshold=0
  Switch1 : Switch  Threshold=eps
  s=s(F/W) : Lookup  InputValues=wh_slip_force_coeff  OutputValues=wh_slip
  vehicle speed (m/s) : Product  Inputs=3  Multiplication=Element-wise(.*)  SaturateOnIntegerOverflow=on
  possible vehicle speed (m/s) : Outport  Port=1  InitialOutput=0
  tag scope: veh_spd_a_rec=global
  wires:
  Product/1 -> Sum3/1
  vehicle speed (m/s)/1 -> [veh_spd_a_rec], Switch1/1
  Switch1/1 -> possible vehicle speed (m/s)/1
  tractive force available at front axle (N)/1 -> Abs/1, Sign/1
  weight borne by front axle (N)/1 -> F/W/2
  Abs1/1 -> Relational Operator1/1
  Constant/1 -> Relational Operator1/2
  axle speed req'd (rad/s)/1 -> Sum4/2
  Sum4/1 -> Abs1/1
  vehicle speed required (m/s)/1 -> Switch1/3
  Relational Operator1/1 -> Switch1/2
  Constant6/1 -> vehicle speed (m/s)/3
  axle speed available (rad/s)/1 -> vehicle speed (m/s)/2, Sum4/1
  s=s(F/W)/1 -> Product/1
  Sign/1 -> Product/2
  F/W/1 -> Switch/1
  Constant5/1 -> Sum3/2
  Fcn/1 -> vehicle speed (m/s)/1
  Sum3/1 -> Fcn/1
  Switch/1 -> Saturation/1
  Saturation/1 -> s=s(F/W)/1
  Abs/1 -> Relational Operator/1, F/W/1
  Relational Operator/1 -> Switch/2
  Constant3/1 -> Relational Operator/2, Switch/3

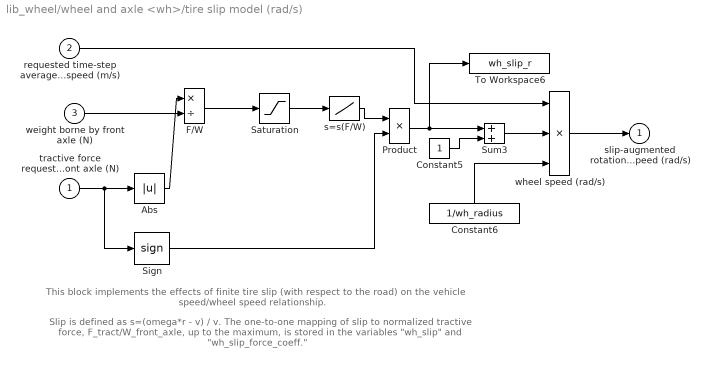
== system lib_wheel/wheel and axle <wh>/tire slip model (rad/s) ==
  note: This block implements the effects of finite tire slip
      | (with respect to the road) on the vehicle speed/wheel speed relationship.
  note: Slip is defined as s=(omega*r - v) / v.  The one-to-one mapping of slip to normalized
      | tractive force, F_tract/W_front_axle, up to the maximum, is stored in the variables
      | "wh_slip" and "wh_slip_force_coeff."
  tractive force requested of front axle (N) : Inport  Port=1  LatchInput=off
  requested time-step average vehicle speed (m/s) : Inport  Port=2  LatchInput=off
  weight borne by front axle (N) : Inport  Port=3  LatchInput=off
  Abs : Abs  SaturateOnIntegerOverflow=on
  Constant5 : Constant  Value=1
  Constant6 : Constant  Orientation=up  Value=1/wh_radius
  F/W : Product  Inputs=*/  Multiplication=Element-wise(.*)  SaturateOnIntegerOverflow=on
  Product : Product  Inputs=2  Multiplication=Element-wise(.*)  SaturateOnIntegerOverflow=on
  Saturation : Saturate  UpperLimit=max(wh_slip_force_coeff)  LowerLimit=min(wh_slip_force_coeff)  LinearizeAsGain=on
  Sign : Signum
  Sum3 : Sum  Inputs=++  SaturateOnIntegerOverflow=on
  To Workspace6 : ToWorkspace  VariableName=wh_slip_r  SampleTime=-1  SaveFormat=Array
  s=s(F/W) : Lookup  InputValues=wh_slip_force_coeff  OutputValues=wh_slip
  wheel speed (rad/s) : Product  Inputs=3  Multiplication=Element-wise(.*)  SaturateOnIntegerOverflow=on
  slip-augmented rotational speed (rad/s) : Outport  Port=1  InitialOutput=0
  wires:
  Product/1 -> To Workspace6/1, Sum3/1
  s=s(F/W)/1 -> Product/1
  wheel speed (rad/s)/1 -> slip-augmented rotational speed (rad/s)/1
  tractive force requested of front axle (N)/1 -> Abs/1, Sign/1
  Constant5/1 -> Sum3/2
  Sum3/1 -> wheel speed (rad/s)/2
  Constant6/1 -> wheel speed (rad/s)/3
  requested time-step average vehicle speed (m/s)/1 -> wheel speed (rad/s)/1
  Sign/1 -> Product/2
  Abs/1 -> F/W/1
  F/W/1 -> Saturation/1
  Saturation/1 -> s=s(F/W)/1
  weight borne by front axle (N)/1 -> F/W/2

== system lib_wheel/wheel and axle <wh>/traction controller interface ==
  F_req : Inport  Port=1  LatchInput=off
  v_ave_req : Inport  Port=2  LatchInput=off
  F_req_limited : Outport  Port=1  InitialOutput=0
  v_req_limited : Outport  Port=2  InitialOutput=0
  wt_front_axle : Outport  Port=3  InitialOutput=0
  tag scope: F_req=global, v_ave_req=global
  wires:
  v_ave_req/1 -> [v_ave_req]
  F_req/1 -> [F_req]
  [wt_front_axle] -> wt_front_axle/1
  [v_req_limited] -> v_req_limited/1
  [F_req_limited] -> F_req_limited/1

== system lib_wheel/wheel and axle  front/rear <wh>/Block NOTES ==
  note: This block determines the required axle torque and speed given the tractive force and
      | speed required to meet the trace in the top blocks, and determines the available tractive
      | force and possible vehicle speed given the drivetrain-input torque and rotational speed
      | in the bottom blocks.  The "wheel control" blocks apply the braking strategy and ensure
      | that accelerations beyond the capability of the tires are not requested.

== system lib_wheel/wheel and axle  front/rear <wh>/effect of  inertia (Nm) ==
  note: This block computes the torque required to overcome the inertia of the
      | wheels and axle.
  axle input speed (rad/s) : Inport  Port=1  LatchInput=off
  Constant : Constant  Value=wh_inertia
  Product : Product  Inputs=2  Multiplication=Element-wise(.*)  SaturateOnIntegerOverflow=on
  d/dt : Derivative
  inertia torque (Nm) : Outport  Port=1  InitialOutput=0
  wires:
  d/dt/1 -> Product/1
  axle input speed (rad/s)/1 -> d/dt/1
  Constant/1 -> Product/2
  Product/1 -> inertia torque (Nm)/1

== system lib_wheel/wheel and axle  front/rear <wh>/front brake ==
  F_brake : Inport  Port=1  LatchInput=off
  Constant : Constant  Value=wh_max_front_brake_force
  Terminator : Terminator
  F_brake_max : Outport  Port=1  InitialOutput=0
  wires:
  F_brake/1 -> Terminator/1
  Constant/1 -> F_brake_max/1

== system lib_wheel/wheel and axle  front/rear <wh>/front force ==
  In1 : Inport  Orientation=up  Port=1  LatchInput=off
  In2 : Inport  Port=2  LatchInput=off
  Product1 : Product  Inputs=2  Multiplication=Element-wise(.*)  SaturateOnIntegerOverflow=on
  Sum2 : Sum  Inputs=-+  SaturateOnIntegerOverflow=on
  To Workspace12 : ToWorkspace  VariableName=wh_front_brake_r  SampleTime=-1  SaveFormat=Array
  brake request  controller interface : Subsystem
      settings: RTWFcnNameOpts=Auto  RTWFileNameOpts=Auto
  tractive torque req/d of drivetrain (Nm) : Gain  Gain=wh_radius  Multiplication=Element-wise(K.*u)  SaturateOnIntegerOverflow=on
  Out1 : Outport  Port=1
  wires:
  brake request  controller interface/1(F_front_brake_req) -> Sum2/1, To Workspace12/1
  Sum2/1 -> tractive torque req/d of drivetrain (Nm)/1
  Product1/1 -> Sum2/2
  In1/1 -> Product1/1
  In2/1 -> Product1/2
  tractive torque req/d of drivetrain (Nm)/1 -> Out1/1

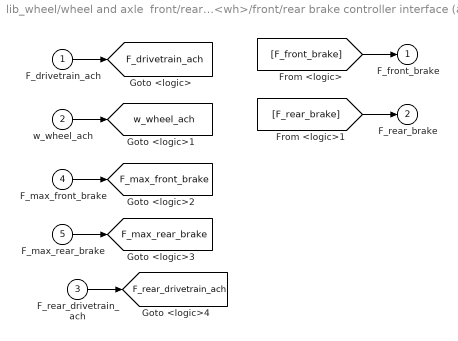
== system lib_wheel/wheel and axle  front/rear <wh>/front/rear brake controller interface (achievable) ==
  F_drivetrain_ach : Inport  Port=1  LatchInput=off
  w_wheel_ach : Inport  Port=2  LatchInput=off
  F_rear_drivetrain_ach : Inport  Port=3  LatchInput=off
  F_max_front_brake : Inport  Port=4  LatchInput=off
  F_max_rear_brake : Inport  Port=5  LatchInput=off
  F_front_brake : Outport  Port=1  InitialOutput=0
  F_rear_brake : Outport  Port=2  InitialOutput=0
  tag scope: F_drivetrain_ach=global, F_max_front_brake=global, F_max_rear_brake=global, F_rear_drivetrain_ach=global, w_wheel_ach=global
  wires:
  [F_rear_brake] -> F_rear_brake/1
  [F_front_brake] -> F_front_brake/1
  w_wheel_ach/1 -> [w_wheel_ach]
  F_drivetrain_ach/1 -> [F_drivetrain_ach]
  F_max_front_brake/1 -> [F_max_front_brake]
  F_max_rear_brake/1 -> [F_max_rear_brake]
  F_rear_drivetrain_ach/1 -> [F_rear_drivetrain_ach]

== system lib_wheel/wheel and axle  front/rear <wh>/help ==

== system lib_wheel/wheel and axle  front/rear <wh>/limits and losses diagnostics ==
  speed : Inport  Orientation=down  Port=1  LatchInput=off
  front brake : Inport  Port=2  LatchInput=off
  front brake max : Inport  Port=3  LatchInput=off
  rear brake max : Inport  Port=4  LatchInput=off
  rear brake : Inport  Port=5  LatchInput=off
  Gain : Gain  Gain=-1  Multiplication=Element-wise(K.*u)  SaturateOnIntegerOverflow=on
  Logical Operator : Logic  Operator=OR  Inputs=2
  Product : Product  Inputs=2  Multiplication=Element-wise(.*)  SaturateOnIntegerOverflow=on
  Relational Operator1 : RelationalOperator  Operator===
  Relational Operator2 : RelationalOperator  Operator===
  Sum3 : Sum  Inputs=++  SaturateOnIntegerOverflow=on
  To Workspace6 : ToWorkspace  VariableName=wh_brake_loss_pwr  SampleTime=-1  SaveFormat=Array
  tag scope: brake_limited=global
  wires:
  Gain/1 -> Product/2
  Sum3/1 -> Gain/1
  Product/1 -> To Workspace6/1
  Logical Operator/1 -> [brake_limited]
  Relational Operator1/1 -> Logical Operator/1
  Relational Operator2/1 -> Logical Operator/2
  speed/1 -> Product/1
  front brake/1 -> Sum3/1, Relational Operator1/1
  front brake max/1 -> Relational Operator1/2
  rear brake max/1 -> Relational Operator2/1
  rear brake/1 -> Sum3/2, Relational Operator2/2

== system lib_wheel/wheel and axle  front/rear <wh>/loss (Nm) ==
  note: The loss torque is zero when the axle is not turning.
  axle speed (rad/s) : Inport  Port=1  LatchInput=off
  Constant : Constant  Orientation=up  Value=0
  Switch : Switch  Threshold=eps
  veh mass calc : lib_wheel/Submodels/veh mass calc
      settings: RTWFcnNameOpts=Auto  RTWFileNameOpts=Auto
  wheel & axle bearing drag (Nm) : Lookup  InputValues=wh_axle_loss_mass  OutputValues=wh_axle_loss_trq
  drag torque (Nm) : Outport  Port=1  InitialOutput=0
  wires:
  veh mass calc/1 -> wheel & axle bearing drag (Nm)/1
  Switch/1 -> drag torque (Nm)/1
  axle speed (rad/s)/1 -> Switch/2
  Constant/1 -> Switch/3
  wheel & axle bearing drag (Nm)/1 -> Switch/1

== system lib_wheel/wheel and axle  front/rear <wh>/rear brake ==
  F_brake : Inport  Port=1  LatchInput=off
  Constant : Constant  Value=wh_max_rear_brake_force
  Terminator : Terminator
  F_brake_max : Outport  Port=1  InitialOutput=0
  wires:
  Constant/1 -> F_brake_max/1
  F_brake/1 -> Terminator/1
